simulink model "nekiprimer"  (R2018a)
settings: Solver=ode4  StartTime=0.0  StopTime=100  FixedStep=0.0001  RelTol=1e-3
settings Model: Creator=Teodor  LastModifiedBy=Teodor

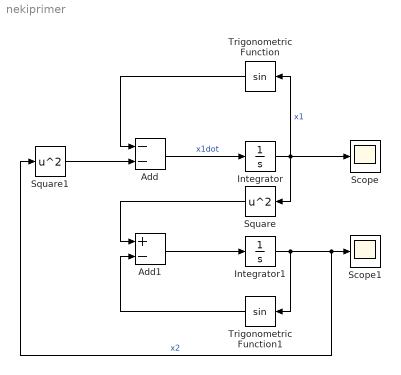
== system nekiprimer ==
  Add : Sum  Inputs=--
  Add1 : Sum  Inputs=+-
  Integrator : Integrator  InitialCondition=[-1:1]
  Integrator1 : Integrator  InitialCondition=[-1:1]
  Scope : Scope
  Scope1 : Scope
  Square : Math  Operator=square  SaturateOnIntegerOverflow=on
  Square1 : Math  Operator=square  SaturateOnIntegerOverflow=on
  Trigonometric Function : Trigonometry
  Trigonometric Function1 : Trigonometry
  wires:
  Add/1 -> Integrator/1  "x1dot"
  Integrator/1 -> Square/1, Scope/1, Trigonometric Function/1  "x1"
  Trigonometric Function/1 -> Add/1
  Integrator1/1 -> Square1/1, Scope1/1, Trigonometric Function1/1  "x2"
  Add1/1 -> Integrator1/1
  Trigonometric Function1/1 -> Add1/2
  Square/1 -> Add1/1
  Square1/1 -> Add/2
